simulink model "lookup_nD_TestGen31"  (R2017b)
settings: Solver=FixedStepDiscrete  StartTime=0.0  StopTime=10.0  RelTol=1e-3
settings Model: Creator=ktrinh  LastModifiedBy=ktrinh
settings DebuggingCC: ParameterOverflowMsg=none

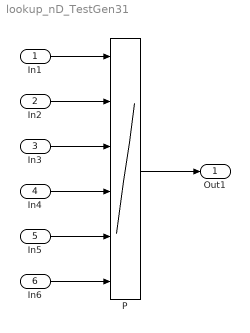
== system lookup_nD_TestGen31 ==
  In1 : Inport  OutMin=0  OutMax=127  OutDataTypeStr=single  PortDimensions=1
  In2 : Inport  Port=2  OutMin=0  OutMax=127  OutDataTypeStr=single
  In3 : Inport  Port=3  OutMin=0  OutMax=127  OutDataTypeStr=single
  In4 : Inport  Port=4  OutMin=0  OutMax=127  OutDataTypeStr=single
  In5 : Inport  Port=5  OutMin=0  OutMax=127  OutDataTypeStr=single
  In6 : Inport  Port=6  OutMin=0  OutMax=127  OutDataTypeStr=single
  P : Lookup_n-D  NumberOfTableDimensions=6  BreakpointsForDimension1=[60.4296403833363;88.3232237593451]  BreakpointsForDimension2=[6.59402580149658;51.7978488623655;62.0261739226904;74.4676694719636;96.7983533783949]  BreakpointsForDimension3=[37.5809884163919;97.499576326139;102.821330151236]  BreakpointsForDimension4=[52.3321686501254;69.0281428704222]  BreakpointsForDimension5=[1.18904504302478;51.2954398690221;56.1261841898742]  BreakpointsForDimension6=[7.62113229658154;32.5872964340294;56.4418548843695;89.9837588331008]  BreakpointsForDimension1DataTypeStr=int16  BreakpointsForDimension2DataTypeStr=int16  BreakpointsForDimension3DataTypeStr=int16  BreakpointsForDimension4DataTypeStr=int16  BreakpointsForDimension5DataTypeStr=int16  BreakpointsForDimension6DataTypeStr=int16  Table=reshape(repmat([4 5 6 7 8;16 19 20 21 22;10 18 23 24 25],6,8),[2,5,3,2,3, 4])  TableDataTypeStr=double  InterpMethod=Flat  ExtrapMethod=Clip  UseLastTableValue=on  InternalRulePriority=Speed  OutDataTypeStr=Inherit: Inherit from 'Table data'  RndMeth=Nearest  SaturateOnIntegerOverflow=on  InputSameDT=on
  Out1 : Outport
  wires:
  In1/1 -> P/1
  In2/1 -> P/2
  In3/1 -> P/3
  In4/1 -> P/4
  In5/1 -> P/5
  In6/1 -> P/6
  P/1 -> Out1/1
